simulink model "SwingTaskNorm"  (R2024b)
settings: Solver=ode45  StartTime=0.0  StopTime=Stoptime  FixedStep=1e-4  MaxStep=1e-3  MinStep=1e-21  RelTol=1e-6  AbsTol=1e-9
values from neighbouring files (symbols this model uses):
  d = 0    [Landscape_SwingTask_Norm.m]    (also in Landscape_SwingTask_Norm.mat)
  dtheta_0 = 0    [Landscape_SwingTask_Norm.m]    (also in Landscape_SwingTask_Norm.mat)
  g = 0    [Landscape_SwingTask_Norm.m]    (also in Landscape_SwingTask_Norm.mat)
  I = 1    [Landscape_SwingTask_Norm.m]    (also in Landscape_SwingTask_Norm.mat)
  inverse = +1    (= 1)    [Landscape_SwingTask_Norm.m]    (also in Landscape_SwingTask_Norm.mat)
  Kd = KDs(i,j)    [Landscape_SwingTask_Norm.m]    (also in Landscape_SwingTask_Norm.mat = 1.3; run_SwingTask_Norm.m = Gains(2))
  Ki = 0    [Landscape_SwingTask_Norm.m]    (also in Landscape_SwingTask_Norm.mat; Master_SwingTask_Norm.m; TisofitST_v13.mat; optGains_SwingTask_Norm.mat)
  Kp = KPs(i,j)    [Landscape_SwingTask_Norm.m]    (also in Landscape_SwingTask_Norm.mat = 0.3; run_SwingTask_Norm.m = Gains(1))
  l = 1    [Landscape_SwingTask_Norm.m]    (also in Landscape_SwingTask_Norm.mat)
  m = 1    [Landscape_SwingTask_Norm.m]    (also in Landscape_SwingTask_Norm.mat)
  t_delay = 1    [Landscape_SwingTask_Norm.m]    (also in Landscape_SwingTask_Norm.mat)
  tau_iso = 1e12    (= 1000000000000)    [Landscape_SwingTask_Norm.m]    (also in Landscape_SwingTask_Norm.mat)
  theta_0 = 0    [Landscape_SwingTask_Norm.m]    (also in Landscape_SwingTask_Norm.mat)
  theta_r = 1    [Landscape_SwingTask_Norm.m]    (also in Landscape_SwingTask_Norm.mat)
settings Model: Creator=C. David Remy  LastModifiedBy=smohamedthangal
settings SolverCC: MaxConsecutiveMinStep=10000  ZeroCrossAlgorithm=Adaptive  AlgebraicLoopSolver=LineSearch
settings DataIOCC: ReturnWorkspaceOutputs=off
settings OptimizationCC: ReuseModelBlockBuffer=off  AccelVerboseBuild=on
settings DebuggingCC: MaskedZcDiagnostic=none  IgnoredZcDiagnostic=none  UnconnectedInputMsg=warning  UnconnectedOutputMsg=warning  UnconnectedLineMsg=warning  ArithmeticOperatorsInVariantConditions=warning
settings ModelReferenceCC: EnableRefExpFcnMdlSchedulingChecks=on
settings SFSimCC: SimUseLocalCustomCode=off  CustomCodeUndefinedFunction=UseInterfaceOnly
settings RTWCC: RTWUseLocalCustomCode=off  GPUComputeCapability=3.5

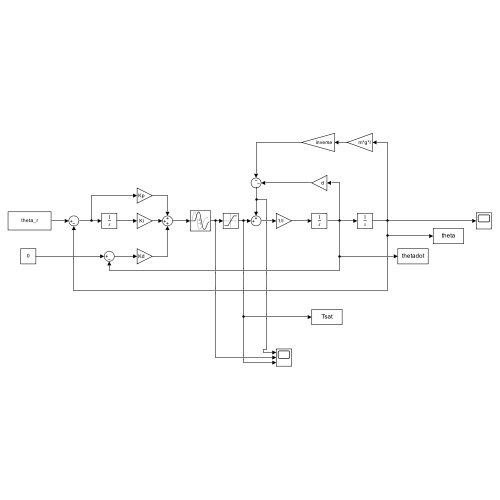
[thumbnail: Simulink's stored preview of the top-level diagram]
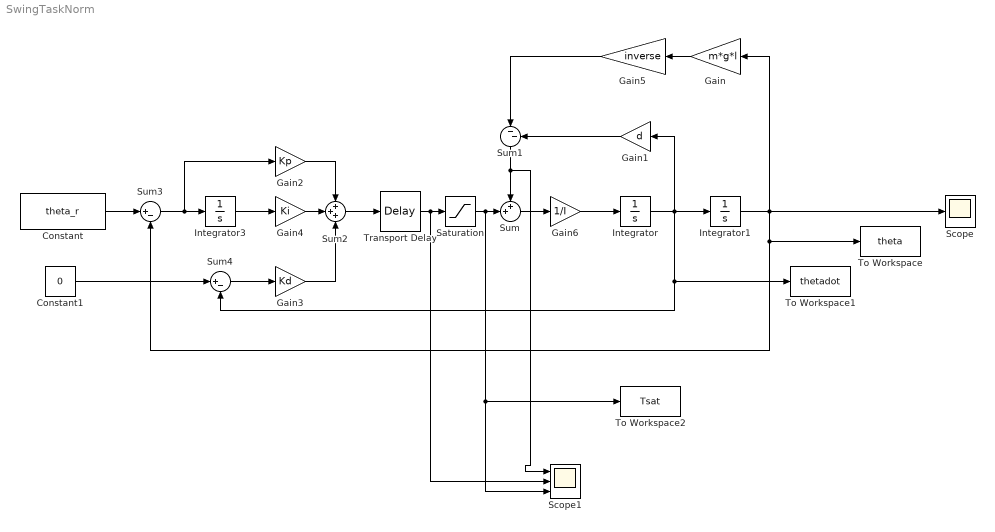
== system SwingTaskNorm ==
  Constant : Constant  Value=theta_r
  Constant1 : Constant  Value=0
  Gain : Gain  Gain=m*g*l
  Gain1 : Gain  Gain=d
  Gain2 : Gain  Gain=Kp
  Gain3 : Gain  Gain=Kd
  Gain4 : Gain  Gain=Ki
  Gain5 : Gain  Gain=inverse
  Gain6 : Gain  Gain=1/I
  Integrator : Integrator  InitialCondition=dtheta_0
  Integrator1 : Integrator  InitialCondition=theta_0
  Integrator3 : Integrator
  Saturation : Saturate  UpperLimit=+tau_iso  LowerLimit=-tau_iso
  Scope : Scope
  Scope1 : Scope  NumInputPorts=3
  Sum : Sum  Inputs=++|
  Sum1 : Sum  Inputs=|--
  Sum2 : Sum  Inputs=+++
  Sum3 : Sum  Inputs=|+-
  Sum4 : Sum  Inputs=|+-
  To Workspace : ToWorkspace  VariableName=theta  SaveFormat=Timeseries  SampleTime=-1
  To Workspace1 : ToWorkspace  VariableName=thetadot  SaveFormat=Timeseries  SampleTime=-1
  To Workspace2 : ToWorkspace  VariableName=Tsat  SaveFormat=Timeseries  SampleTime=-1
  Transport Delay : TransportDelay  DelayTime=t_delay
  wires:
  Integrator/1 -> Sum4/2, To Workspace1/1, Gain1/1, Integrator1/1
  Sum/1 -> Gain6/1
  Gain/1 -> Gain5/1
  Gain1/1 -> Sum1/2
  Gain5/1 -> Sum1/1
  Saturation/1 -> Sum/2, To Workspace2/1, Scope1/3
  Transport Delay/1 -> Scope1/2, Saturation/1
  Sum2/1 -> Transport Delay/1
  Sum1/1 -> Sum/1, Scope1/1
  Integrator3/1 -> Gain4/1
  Gain4/1 -> Sum2/2
  Gain3/1 -> Sum2/3
  Gain2/1 -> Sum2/1
  Sum4/1 -> Gain3/1
  Constant/1 -> Sum3/1
  Constant1/1 -> Sum4/1
  Sum3/1 -> Gain2/1, Integrator3/1
  Gain6/1 -> Integrator/1
  Integrator1/1 -> Sum3/2, To Workspace/1, Scope/1, Gain/1
